simulink model "untitled"  (R2024b)
settings: Solver=VariableStepAuto  StartTime=0.0  StopTime=10.0  RelTol=1e-3
settings Model: Creator=robin  LastModifiedBy=robin

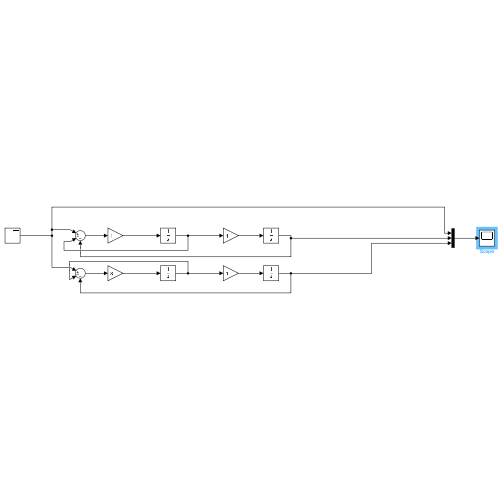
[thumbnail: Simulink's stored preview of the top-level diagram]
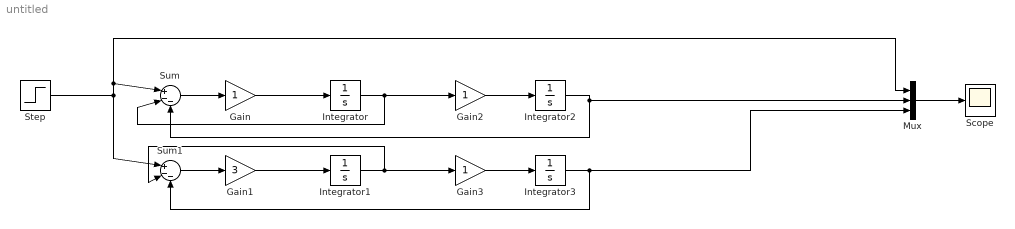
== system untitled ==
  Gain : Gain
  Gain1 : Gain  Gain=3
  Gain2 : Gain
  Gain3 : Gain
  Integrator{,1..3} (4 alike) : Integrator
  Mux : Mux  Inputs=3
  Scope : Scope
  Step : Step  SampleTime=0
  Sum : Sum  Inputs=|+--
  Sum1 : Sum  Inputs=|+--
  wires:
  Step/1 -> Mux/1, Sum/1, Sum1/1
  Gain/1 -> Integrator/1
  Gain1/1 -> Integrator1/1
  Integrator/1 -> Gain2/1, Sum/2
  Sum/1 -> Gain/1
  Sum1/1 -> Gain1/1
  Mux/1 -> Scope/1
  Integrator1/1 -> Sum1/2, Gain3/1
  Gain3/1 -> Integrator3/1
  Gain2/1 -> Integrator2/1
  Integrator2/1 -> Mux/2, Sum/3
  Integrator3/1 -> Mux/3, Sum1/3
